simulink model "synchro"  (R2020b)
settings: Solver=FixedStepDiscrete  StartTime=0.0  StopTime=0.01  RelTol=1e-3
libraries: simulink x1
Description:
  | This model uses Universal Software Radio Peripheral (USRP) hardware with Simulink(R) to perform FM demodulation and stereo decoding.
settings Model: Creator=druffle  LastModifiedBy=druffle
settings DataIOCC: SaveFormat=Structure  SaveOutput=off  SignalLogging=off  DSMLogging=off  SaveTime=off  ReturnWorkspaceOutputs=off
settings OptimizationCC: ExpressionDepthLimit=2147483647  EfficientMapNaN2IntZero=off  LifeSpan=inf  SimCompilerOptimization=on
settings DebuggingCC: UnderspecifiedInitializationDetection=Classic  MergeDetectMultiDrivingBlocksExec=none  SolverPrmCheckMsg=warning  InheritedTsInSrcMsg=none  MultiTaskCondExecSysMsg=none  ParameterPrecisionLossMsg=none  FcnCallInpInsideContextMsg=warning  AllowSymbolicDim=off  StateNameClashWarn=warning  SFUnexpectedBacktrackingDiag=warning  SFNoUnconditionalDefaultTransitionDiag=warning  SFExecutionAtInitializationDiag=none  ArithmeticOperatorsInVariantConditions=warning
settings HardwareCC: ProdBitPerPointer=32  ProdBitPerSizeT=32  ProdBitPerPtrDiffT=32  ProdLargestAtomicFloat=None  ProdIntDivRoundTo=Undefined  ProdEndianess=Unspecified  ProdWordSize=32  ProdHWDeviceType=32-bit Generic  TargetBitPerPointer=64  TargetBitPerSizeT=64  TargetBitPerPtrDiffT=64  TargetLongLongMode=on  TargetIntDivRoundTo=Zero  TargetEndianess=LittleEndian  TargetWordSize=64  TargetHWDeviceType=Generic->MATLAB Host Computer  ProdEqTarget=off
settings ModelReferenceCC: PropagateSignalLabelsOutOfModel=off
settings SFSimCC: SimIntegrity=off  SimUseLocalCustomCode=off  CustomCodeUndefinedFunction=UseInterfaceOnly
settings RTWCC: RTWUseLocalCustomCode=off
settings RTWCC: CustomSourceCode=|
  | #include <stdio.h>
  | #include <stdlib.h>
settings CodeAppCC: MaxIdLength=128  StateflowObjectComments=on
settings GRTTargetCC: TargetLangStandard=C89/C90 (ANSI)  CombineOutputUpdateFcns=off  GRTInterface=on
settings ConfigComp: CovMetricSettings=dw  CovSaveCumulativeToWorkspaceVar=on  CovSaveSingleToWorkspaceVar=on  CovExternalEMLEnable=off  CovSFcnEnable=off

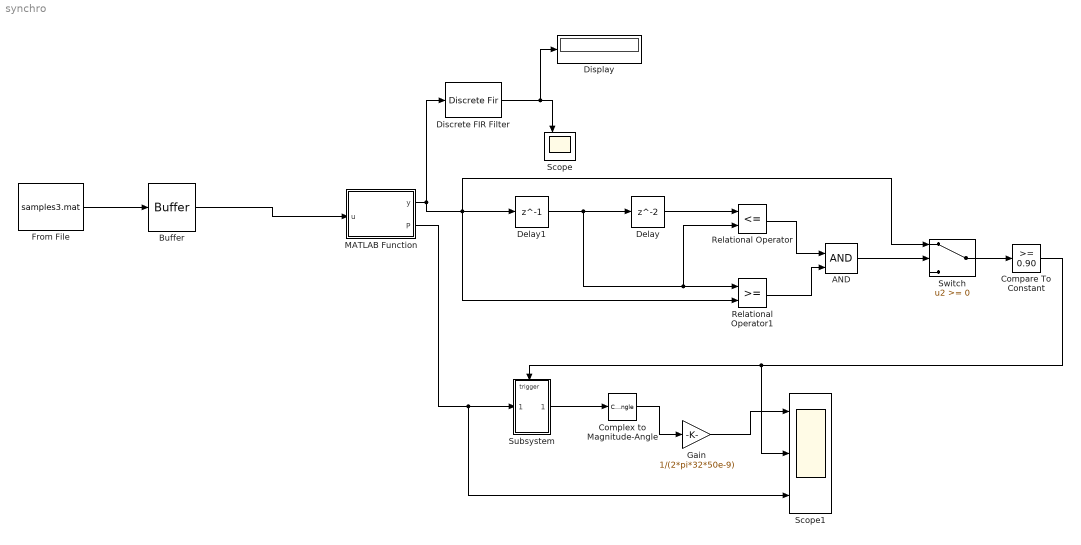
== system synchro ==
  AND : Logic  IconShape=distinctive  AllPortsSameDT=off  OutDataTypeStr=boolean
  Buffer : Buffer  V=63  OutputFrames=off
  Compare To Constant : simulink/Logic and Bit Operations/Compare To Constant  relop=>=  const=0.90  OutDataTypeStr=boolean
  Complex to Magnitude-Angle : ComplexToMagnitudeAngle  Output=Angle
  Delay : Delay
  Delay1 : Delay  DelayLength=1
  Discrete FIR Filter : DiscreteFir  Coefficients=[1/3 1/3 1/3]
  Display : Display
  From File : FromFile  FileName=samples3.mat  SampleTime=50e-9  ExtrapolationAfterLastDataPoint=Ground value
  Gain : Gain  Gain=1/(2*pi*32*50e-9)
  MATLAB Function : MATLAB Function  TreatAsAtomicUnit=on
  Relational Operator : RelationalOperator  Operator=<=  OutDataTypeStr=boolean  RndMeth=Simplest
  Relational Operator1 : RelationalOperator  OutDataTypeStr=boolean  RndMeth=Simplest
  Scope : Scope  NumInputPorts=2
  Scope1 : Scope  NumInputPorts=3
  Subsystem : Subsystem
  Switch : Switch
  wires:
  From File/1 -> Buffer/1
  Buffer/1 -> MATLAB Function/1(u)
  MATLAB Function/1(y) -> Switch/1, Relational Operator1/2, Delay1/1, Discrete FIR Filter/1
  Discrete FIR Filter/1 -> Display/1, Scope/1
  Delay1/1 -> Relational Operator/2, Relational Operator1/1, Delay/1
  Relational Operator/1 -> AND/1
  Relational Operator1/1 -> AND/2
  AND/1 -> Switch/2
  Delay/1 -> Relational Operator/1
  Gain/1 -> Scope1/1
  Switch/1 -> Compare To Constant/1
  MATLAB Function/2(P) -> Scope1/3, Subsystem/1(In1)
  Compare To Constant/1 -> Subsystem/Trigger, Scope1/2
  Subsystem/1(Out1) -> Complex to Magnitude-Angle/1
  Complex to Magnitude-Angle/1 -> Gain/1

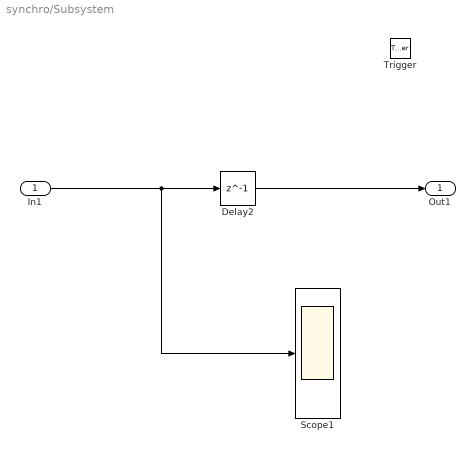
== system synchro/Subsystem ==
  In1 : Inport
  Trigger : TriggerPort  VariantControl=Variant  PortDimensions=1
  Delay2 : Delay  DelayLength=1
  Scope1 : Scope
  Out1 : Outport
  wires:
  In1/1 -> Scope1/1, Delay2/1
  Delay2/1 -> Out1/1

== matlab function synchro/MATLAB Function ==
  data: u input; y output; P output
function [y, P]= fcn(u)

    L = 32;

    samples = u;
    t = length(samples);
    T = 64*50e-9;
    start = 1;
    Ng = 3;
    ds = 1;
    d=0;

    % Initialiser à zéro
    %phi = zeros(1, uint64((t/(2*L))+1));
    %res=zeros(1, uint64((t/(2*L))+1));
        % calculer la corrélation entre les échantillons d et d+L
        P = sum(samples(d+L+1:d+L+L) .* conj(samples(d+1:d+L)));
        % normaliser la corrélation par l'énergie du demi-symbole
        R = sum(abs(samples(d+1+L:d+L+L)).^2);
        Rf=(1/2)*(sum(abs(samples(d:d+63).^2)));
        % vérifier que corr et energy ne sont pas égaux à zéro
        if P ~= 0 && R ~= 0
            M = abs(P).^2 ./ R.^2;
        else
            M = 0;
        end
        if P~=0 && Rf ~=0
             Mf = abs(P).^2 ./ Rf.^2;
        else
             Mf = 0;
        end

   
       
    


    

y = Mf;
